simulink model "NonLinear_Nomoto2"  (R2015b)
settings: Solver=VariableStepAuto  StartTime=0.0  StopTime=tstop  FixedStep=0.01  RelTol=1e-3
values from neighbouring files (symbols this model uses):
  b_1 = [800009.963225 12.8568262477]    [H_b_curvefitting.mat]    (also in Yaw and Yaw-rate controller.mat = [800009.882282 13.5298731691]; Yaw_NonLin_controller.mat; analyse_ulin_dynamics kopi.m = lsqcurvefit(F5, b_1_0, r_list_c, d_list,[],[],OPT); analyse_ulin_dynamics.m = lsqcurvefit(F5, b_1_0, r_list_c, d_list,[1e5 0],[inf inf],OP)
  delta_c = dc_list(i)    [NonLinearAnalysis.m]    (also in Run_Delta_R_Sim.m = d_list(i); analyse_lin_dynamics.m = deg2rad(delta_list(i)); analyse_ulin_dynamics kopi.m = deg2rad(delta); analyse_ulin_dynamics.m = deg2rad(delta_list(i)))
  K = 0.0516730310612    [Heading_model.mat]    (also in Nomoto2_curvefitting.mat = 0.0627494534487; analyse_controller.m = place(A,B,P); analyse_lin_dynamics.m = x(2); analyse_ulin_dynamics kopi.m = x(2))
  T1 = 147.34337747    [Heading_model.mat]    (also in Nomoto2_curvefitting.mat = 53.2599278148; analyse_controller.m = 130; analyse_lin_dynamics.m = x(1); analyse_ulin_dynamics kopi.m = x(1))
  T2 = 157.062217136    [Heading_model.mat]    (also in Nomoto2_curvefitting.mat = 67.2891048935; analyse_controller.m = 150; analyse_lin_dynamics.m = x(2); analyse_ulin_dynamics kopi.m = x(2))
  tsamp = 10    [NonLinearAnalysis.m]    (also in analyse_lin_dynamics.m; analyse_steadystate.m; analyse_ulin_dynamics kopi.m; analyse_ulin_dynamics.m)
undefined symbols (not defined in the file or in its folder): b_3
settings Model: Creator=Erik  LastModifiedBy=Erik
settings HardwareCC: ProdBitPerPointer=32  ProdLargestAtomicFloat=None  ProdIntDivRoundTo=Undefined  ProdEndianess=Unspecified  ProdWordSize=32  ProdHWDeviceType=32-bit Generic
settings GRTTargetCC: GeneratePreprocessorConditionals=Disable all

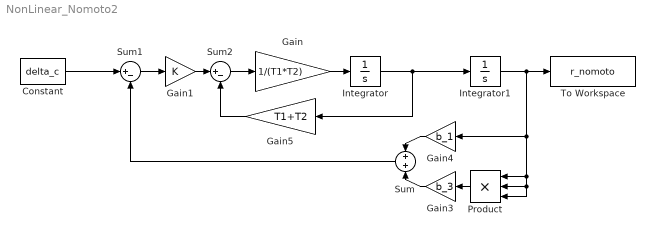
== system NonLinear_Nomoto2 ==
  Constant : Constant  Value=delta_c
  Gain : Gain  Gain=1/(T1*T2)
  Gain1 : Gain  Gain=K
  Gain3 : Gain  Gain=b_3
  Gain4 : Gain  Gain=b_1
  Gain5 : Gain  Gain=T1+T2
  Integrator : Integrator
  Integrator1 : Integrator
  Product : Product  Inputs=3
  Sum : Sum
  Sum1 : Sum  Inputs=|+-
  Sum2 : Sum  Inputs=|+-
  To Workspace : ToWorkspace  VariableName=r_nomoto  SampleTime=tsamp
  wires:
  Integrator/1 -> Gain5/1, Integrator1/1
  Product/1 -> Gain3/1
  Integrator1/1 -> To Workspace/1, Product/3, Product/2, Product/1, Gain4/1
  Gain/1 -> Integrator/1
  Constant/1 -> Sum1/1
  Sum1/1 -> Gain1/1
  Gain3/1 -> Sum/2
  Gain4/1 -> Sum/1
  Sum/1 -> Sum1/2
  Gain1/1 -> Sum2/1
  Sum2/1 -> Gain/1
  Gain5/1 -> Sum2/2
